simulink model "lqr_lin"  (R2024b)
settings: Solver=VariableStepAuto  StartTime=0.0  StopTime=params.simtime  RelTol=1e-3
values from neighbouring files (symbols this model uses):
  params = parameters()    [lqr_STM_compare.m]    (also in lqr_compare.m; lqr_main_isolated.m)
undefined symbols (not defined in the file or in its folder): lin_model
settings Model: Creator=ben83  LastModifiedBy=ben
settings RTWCC: GPUComputeCapability=3.5

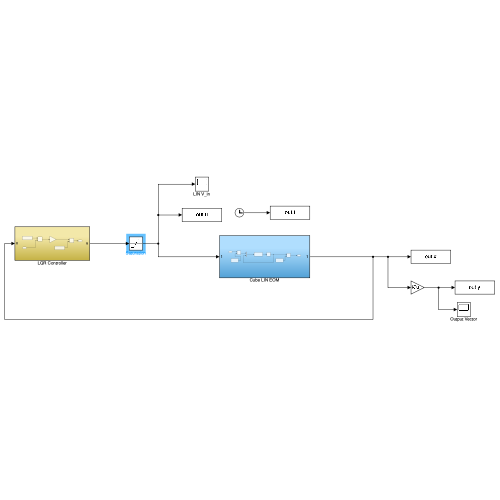
[thumbnail: Simulink's stored preview of the top-level diagram]
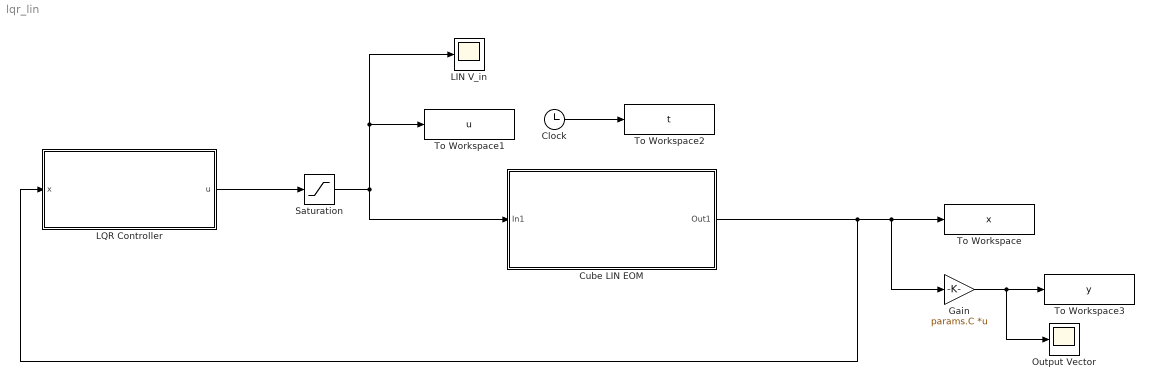
== system lqr_lin ==
  Clock : Clock
  Cube LIN EOM : Subsystem
  Gain : Gain  Gain=params.C  Multiplication=Matrix(K*u)
  LIN V_in : Scope
  LQR Controller : Subsystem
  Output Vector : Scope
  Saturation : Saturate  UpperLimit=10.8  LowerLimit=-10.8
  To Workspace : ToWorkspace  VariableName=x  SampleTime=-1
  To Workspace1 : ToWorkspace  VariableName=u  SampleTime=-1
  To Workspace2 : ToWorkspace  VariableName=t  SampleTime=-1
  To Workspace3 : ToWorkspace  VariableName=y  SampleTime=-1
  wires:
  Clock/1 -> To Workspace2/1
  Saturation/1 -> Cube LIN EOM/1(In1), LIN V_in/1, To Workspace1/1
  LQR Controller/1(u) -> Saturation/1
  Cube LIN EOM/1(Out1) -> LQR Controller/1(x), Gain/1, To Workspace/1
  Gain/1 -> Output Vector/1, To Workspace3/1

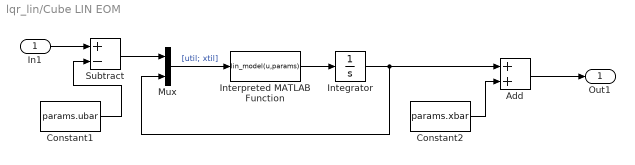
== system lqr_lin/Cube LIN EOM ==
  In1 : Inport
  Add : Sum
  Constant1 : Constant  Value=params.ubar
  Constant2 : Constant  Value=params.xbar
  Integrator : Integrator  InitialCondition=params.iclin
  Interpreted MATLAB Function : MATLABFcn  MATLABFcn=lin_model(u,params)
  Mux : Mux  Inputs=2
  Subtract : Sum  Inputs=+-
  Out1 : Outport
  wires:
  Constant1/1 -> Subtract/2
  Subtract/1 -> Mux/1
  Constant2/1 -> Add/2
  Add/1 -> Out1/1
  In1/1 -> Subtract/1
  Interpreted MATLAB Function/1 -> Integrator/1
  Mux/1 -> Interpreted MATLAB Function/1  "[util; xtil]"
  Integrator/1 -> Add/1, Mux/2

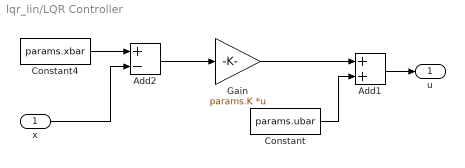
== system lqr_lin/LQR Controller ==
  x : Inport
  Add1 : Sum
  Add2 : Sum  Inputs=+-
  Constant : Constant  Value=params.ubar
  Constant4 : Constant  Value=params.xbar
  Gain : Gain  Gain=params.K  Multiplication=Matrix(K*u)
  u : Outport
  wires:
  x/1 -> Add2/2
  Add1/1 -> u/1
  Constant/1 -> Add1/2
  Gain/1 -> Add1/1
  Constant4/1 -> Add2/1
  Add2/1 -> Gain/1
